simulink model "FilterDesigner"  (R2018b)
settings: Solver=VariableStepAuto  StartTime=0.0  StopTime=4000  RelTol=1e-3
PreLoadFcn:
  | Init
StopFcn:
  | FilterCheck
values from neighbouring files (symbols this model uses):
  fc = 0.33    [Init.m]
  h_win = blackman(N)    [Init.m]
  N = 101    [Init.m]
  NFFT = 1024    [Init.m]
  output_wlength = 24    [Init.m]
undefined symbols (not defined in the file or in its folder): AXI4, bitrevorder, int, Lite
libraries: xbsIndex_r4 x64
settings Model: Creator=joshua goldsmith  LastModifiedBy=jng
settings DebuggingCC: LibraryContextMissingDiagnostic=none
settings SFSimCC: SimUseLocalCustomCode=off
settings RTWCC: RTWUseLocalCustomCode=off

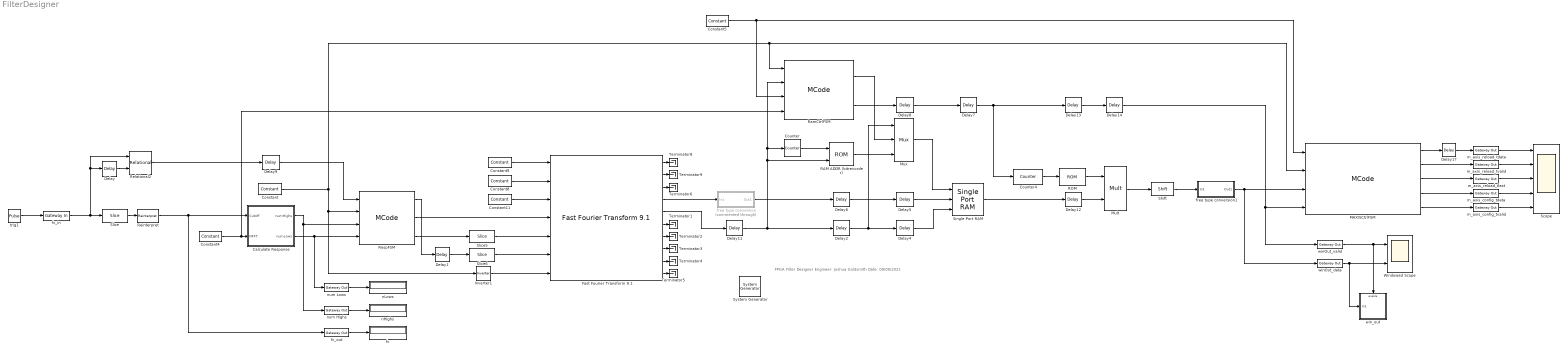
== system FilterDesigner ==
  note: FPGA Filter Designer
      | Engineer: Joshua Goldsmith
      | Date: 09/09/2021
  " System Generator" : xbsIndex_r4/ System Generator  Tag=genX  xilinxfamily=zynq  part=xc7z020  speed=-2  package=clg484  synthesis_tool=Vivado  clock_wrapper=Clock Enables  directory=./iprepo  proj_type=Vivado  Synth_file=Vivado Synthesis Defaults  Impl_file=Vivado Implementation Defaults  testbench=off  simulink_period=1  sysclk_period=10  dcm_input_clock_period=10  incr_netlist=off  trim_vbits=Everywhere in SubSystem  dbl_ovrd=According to Block Masks  core_generation=According to Block Masks  run_coregen=off  deprecated_control=off  eval_field=0  block_type=sysgen
  Calculate Response : Subsystem
  Constant : xbsIndex_r4/Constant  const=0  gui_display_data_type=Boolean  arith_type=Boolean  n_bits=16  bin_pt=14  preci_type=Single  exp_width=8  frac_width=24  explicit_period=on  period=1  equ=P=C  opselect=C  inp2=PCIN>>17  opr=+  inp1=P  carry=CIN  dbl_ovrd=off  block_type=constant
  Constant11 : xbsIndex_r4/Constant  const=0  gui_display_data_type=Fixed-point  arith_type=Signed (2's comp)  n_bits=wlength  bin_pt=flength  preci_type=Single  exp_width=8  frac_width=24  explicit_period=on  period=1  equ=P=C  opselect=C  inp2=PCIN>>17  opr=+  inp1=P  carry=CIN  dbl_ovrd=off  block_type=constant
  Constant4 : xbsIndex_r4/Constant  const=NFFT  gui_display_data_type=Fixed-point  arith_type=Unsigned  n_bits=log2(NFFT)+1  bin_pt=0  preci_type=Single  exp_width=8  frac_width=24  explicit_period=on  period=1  equ=P=C  opselect=C  inp2=PCIN>>17  opr=+  inp1=P  carry=CIN  dbl_ovrd=off  block_type=constant
  Constant5 : xbsIndex_r4/Constant  const=(N-1)/2  gui_display_data_type=Fixed-point  arith_type=Unsigned  n_bits=32  bin_pt=0  preci_type=Single  exp_width=8  frac_width=24  explicit_period=on  period=1  equ=P=C  opselect=C  inp2=PCIN>>17  opr=+  inp1=P  carry=CIN  dbl_ovrd=off  block_type=constant
  Constant8 : xbsIndex_r4/Constant  const=1  gui_display_data_type=Boolean  arith_type=Boolean  n_bits=wlength  bin_pt=flength  preci_type=Single  exp_width=8  frac_width=24  explicit_period=on  period=1  equ=P=C  opselect=C  inp2=PCIN>>17  opr=+  inp1=P  carry=CIN  dbl_ovrd=off  block_type=constant
  Constant9 : xbsIndex_r4/Constant  const=0  gui_display_data_type=Fixed-point  arith_type=Unsigned  n_bits=1  bin_pt=0  preci_type=Single  exp_width=8  frac_width=24  explicit_period=on  period=1  equ=P=C  opselect=C  inp2=PCIN>>17  opr=+  inp1=P  carry=CIN  dbl_ovrd=off  block_type=constant
  Counter : xbsIndex_r4/Counter  cnt_type=Free Running  cnt_to=Inf  operation=Up  start_count=0  cnt_by_val=1  arith_type=Unsigned  n_bits=log2(NFFT)  bin_pt=0  load_pin=off  rst=off  en=on  explicit_period=on  period=1  use_behavioral_HDL=off  implementation=Fabric  dbl_ovrd=off  block_type=counter
  Counter4 : xbsIndex_r4/Counter  cnt_type=Count Limited  cnt_to=size(h_win(1:size(h_win,1)/2+1),1)-1  operation=Up  start_count=0  cnt_by_val=1  arith_type=Unsigned  n_bits=ceil(log2(N/2))  bin_pt=0  load_pin=off  rst=off  en=on  explicit_period=on  period=1  use_behavioral_HDL=off  implementation=Fabric  dbl_ovrd=off  block_type=counter
  Delay{,2,4,6..8,11..14,17} (11 alike) : xbsIndex_r4/Delay  rst=off  infoeditControl=Selection of Reset will increase slice count due to use of real FFs and instead of SRLs  en=off  latency=1  reg_retiming=off  dbl_ovrd=off  block_type=delay
  Delay1 : xbsIndex_r4/Delay  rst=off  infoeditControl=Selection of Reset will increase slice count due to use of real FFs and instead of SRLs  en=off  latency=NFFT-1  reg_retiming=off  dbl_ovrd=off  block_type=delay
  Delay5 : xbsIndex_r4/Delay  rst=off  infoeditControl=Selection of Reset will increase slice count due to use of real FFs and instead of SRLs  en=off  latency=2  reg_retiming=off  dbl_ovrd=off  block_type=delay
  Delay9 : xbsIndex_r4/Delay  rst=off  infoeditControl=Selection of Reset will increase slice count due to use of real FFs and instead of SRLs  en=off  latency=3  reg_retiming=off  dbl_ovrd=off  block_type=delay
  "Fast Fourier Transform 9.1 " : xbsIndex_r4/Fast Fourier Transform 9.1   transform_length=1024  target_clock_frequency=100  target_data_throughput=50  implementation_options=pipelined_streaming_io  run_time_configurable_transform_length=off  phase_factor_width=16  scaling_options=unscaled  rounding_modes=truncation  aclken=off  aresetn=on  output_ordering=bit_reversed_order  cyclic_prefix_insertion=off  throttle_scheme=realtime  xk_index=off  ovflo=off  trim_axipin_name=on  memory_options_data=block_ram  memory_options_phase_factors=block_ram  number_of_stages_using_block_ram_for_data_and_phase_factors=2  memory_options_reorder=block_ram  memory_options_hybrid=off  complex_mult_type=use_mults_resources  butterfly_type=use_luts  simulation_type=hybrid_sim  simulation_model=sysgen:xfftv9_cmodel  data_path_portlist={ 's_axis_data_tdata', 'm_axis_data_tdata', 'm_axis_status_tdata', 'event_fft_overflow' }  channels=1  input_ordering=natural_order  input_width=16  ip_name=Fast Fourier Transform  ip_version=9.1  dsptool_ready=true  ipcore_usecache=true  ipcore_useipmodelcache=true  wrapper_available=true  port_translation_map={ 'aclken' => 'en', 'aresetn' => 'rst'}  data_format=fixed_point  block_type=xfft_v9_1
  Inverter1 : xbsIndex_r4/Inverter  en=off  latency=0  dbl_ovrd=off  block_type=inv
  MAXISCtrlFSM : xbsIndex_r4/MCode  mfname=MAXISCtrlFSM  explicit_period=on  period=1  inputsTable={'boundInpExpr'=>['',''],'inputs'=>['x','y']}  outputsTable={'outputs'=>['z'],'suppressOut'=>['off']}  enable_stdout=off  enable_debug=off  suppress_output=on  defparams={}  hide_port_list={}  dbl_ovrd=off  block_type=mcode
  Mult : xbsIndex_r4/Mult  precision=Full  arith_type="Signed  (2's comp)"  n_bits=16  bin_pt=14  quantization=Truncate  overflow=Wrap  en=off  latency=1  use_behavioral_HDL=off  opt=Speed  use_embedded=on  optimum_pipeline=off  pipeline=on  dbl_ovrd=off  use_rpm=on  placement_style=Triangular  block_type=mult
  Mux : xbsIndex_r4/Mux  inputs=2  en=off  latency=1  precision=Full  arith_type=Unsigned  n_bits=16  bin_pt=14  quantization=Truncate  overflow=Wrap  dbl_ovrd=off  block_type=mux
  RAM ADDR (bitrevorder) : xbsIndex_r4/ROM  depth=NFFT  initVector=bitrevorder(0:NFFT-1)  distributed_mem=Block RAM  rst=off  init_reg=0  en=on  latency=1  gui_display_data_type=Fixed-point  arith_type=Unsigned  n_bits=log2(NFFT)  bin_pt=0  preci_type=Single  exp_width=8  frac_width=24  optimize=Area  use_rpm=on  dbl_ovrd=off  block_type=sprom
  ROM : xbsIndex_r4/ROM  depth=(N+1)/2  initVector=h_win(1:size(h_win,1)/2+1)  distributed_mem=Block RAM  rst=off  init_reg=0  en=off  latency=1  gui_display_data_type=Fixed-point  arith_type="Signed  (2's comp)"  n_bits=16  bin_pt=14  preci_type=Single  exp_width=8  frac_width=24  optimize=Area  use_rpm=on  dbl_ovrd=off  block_type=sprom
  RamCtrlFSM : xbsIndex_r4/MCode  mfname=RamCtrlFSM  explicit_period=on  period=1  inputsTable={'boundInpExpr'=>['','','','',''],'inputs'=>['rst','valid_in','M','NFFT','wlength']}  outputsTable={'outputs'=>['addr','valid_out'],'suppressOut'=>['off','off']}  enable_stdout=off  enable_debug=off  suppress_output=on  defparams={}  hide_port_list={}  dbl_ovrd=off  block_type=mcode
  Reinterpret : xbsIndex_r4/Reinterpret  force_arith_type=on  arith_type=Unsigned  force_bin_pt=on  bin_pt=10  block_type=reinterpret
  Relational2 : xbsIndex_r4/Relational  mode=a!=b  op_type=Bool  en=off  latency=0  dbl_ovrd=off  block_type=relational
  RespFSM : xbsIndex_r4/MCode  mfname=RespFSM  explicit_period=on  period=1  inputsTable={'boundInpExpr'=>['','','',''],'inputs'=>['trig','rst','numHighs','numLows']}  outputsTable={'outputs'=>['sof','rout','valid'],'suppressOut'=>['off','off','off']}  enable_stdout=off  enable_debug=off  suppress_output=on  defparams={}  hide_port_list={}  dbl_ovrd=off  block_type=mcode
  Scope : Scope  NumInputPorts=5
  Shift : xbsIndex_r4/Shift  shift_dir=Left  shift_bits=3  en=off  latency=0  precision=Full  arith_type="Signed  (2's comp)"  n_bits=16  bin_pt=14  quantization=Truncate  overflow=Wrap  dbl_ovrd=off  block_type=shift
  Single Port RAM : xbsIndex_r4/Single Port RAM  depth=NFFT  initVector=zeros(1,NFFT)  distributed_mem=Block RAM  write_mode=No Read On Write  rst=off  init_reg=0  en=off  latency=1  optimize=Area  dbl_ovrd=off  block_type=spram
  Slice : xbsIndex_r4/Slice  nbits=10  boolean_output=off  mode=Lower Bit Location + Width  bit1=0  base1=MSB of Input  bit0=0  base0=LSB of Input  dbl_ovrd=off  block_type=slice
  Slice5 : xbsIndex_r4/Slice  nbits=1  boolean_output=on  mode=Lower Bit Location + Width  bit1=0  base1=MSB of Input  bit0=0  base0=LSB of Input  dbl_ovrd=off  block_type=slice
  Slice6 : xbsIndex_r4/Slice  nbits=1  boolean_output=on  mode=Lower Bit Location + Width  bit1=0  base1=MSB of Input  bit0=0  base0=LSB of Input  dbl_ovrd=off  block_type=slice
  Terminator{1..6,8..9} (8 alike) : Terminator
  Windowed Scope : Scope  NumInputPorts=2
  fc : Display
  fc_in : xbsIndex_r4/Gateway In  gui_display_data_type=Fixed-point  arith_type=Unsigned  n_bits=32  bin_pt=0  preci_type=Single  exp_width=8  frac_width=24  rows=1  columns=1  quantization=Truncate  overflow=Wrap  period=1  UseAsADC=off  ADCChannel='1'  interface=AXI4-Lite  automatic_assignment=off  address_offset=12  intf_name=''  intf_description=''  default_value=0  timing_constraint=None  locs_specified=off  LOCs={}  io_standard={}  inherit_from_input=off  hdl_port=on  dbl_ovrd=off  block_type=gatewayin
  fc_out : xbsIndex_r4/Gateway Out  inherit_from_input=off  hdl_port=off  rows=1  columns=1  UseAsDAC=off  DACChannel='1'  interface=None  automatic_assignment=on  address_offset=hex2dec('00')  intf_name=''  intf_description=''  timing_constraint=None  locs_specified=off  LOCs={}  io_standard={}  block_type=gatewayout
  free type conversion : Subsystem  Commented=through  mask{Wordlength=16, FracBit=15}
      mask prompts: FracBit "Fractional Bit Position"
      mask DialogControl DescGroupVar Prompt: Type Conversion
      mask DialogControl DescTextVar Prompt: Select wordlength and fractional bit position
  free type conversion1 : Subsystem  mask{Wordlength=output_wlength, FracBit=output_wlength-1}
      mask prompts: FracBit "Fractional Bit Position"
      mask DialogControl DescGroupVar Prompt: Type Conversion
      mask DialogControl DescTextVar Prompt: Select wordlength and fractional bit position
  m_axis_config_tdata : xbsIndex_r4/Gateway Out  inherit_from_input=off  hdl_port=on  rows=1  columns=1  UseAsDAC=off  DACChannel='1'  interface=None  automatic_assignment=on  address_offset=hex2dec('00')  intf_name=''  intf_description=''  timing_constraint=None  locs_specified=off  LOCs={}  io_standard={}  block_type=gatewayout
  m_axis_config_tvalid : xbsIndex_r4/Gateway Out  inherit_from_input=off  hdl_port=on  rows=1  columns=1  UseAsDAC=off  DACChannel='1'  interface=None  automatic_assignment=on  address_offset=hex2dec('00')  intf_name=''  intf_description=''  timing_constraint=None  locs_specified=off  LOCs={}  io_standard={}  block_type=gatewayout
  m_axis_reload_tdata : xbsIndex_r4/Gateway Out  inherit_from_input=off  hdl_port=on  rows=1  columns=1  UseAsDAC=off  DACChannel='1'  interface=None  automatic_assignment=on  address_offset=hex2dec('00')  intf_name=''  intf_description=''  timing_constraint=None  locs_specified=off  LOCs={}  io_standard={}  block_type=gatewayout
  m_axis_reload_tlast : xbsIndex_r4/Gateway Out  inherit_from_input=off  hdl_port=on  rows=1  columns=1  UseAsDAC=off  DACChannel='1'  interface=None  automatic_assignment=on  address_offset=hex2dec('00')  intf_name=''  intf_description=''  timing_constraint=None  locs_specified=off  LOCs={}  io_standard={}  block_type=gatewayout
  m_axis_reload_tvalid : xbsIndex_r4/Gateway Out  inherit_from_input=off  hdl_port=on  rows=1  columns=1  UseAsDAC=off  DACChannel='1'  interface=None  automatic_assignment=on  address_offset=hex2dec('00')  intf_name=''  intf_description=''  timing_constraint=None  locs_specified=off  LOCs={}  io_standard={}  block_type=gatewayout
  nHighs : Display
  nLows : Display
  "num Highs " : xbsIndex_r4/Gateway Out  inherit_from_input=off  hdl_port=off  rows=1  columns=1  UseAsDAC=off  DACChannel='1'  interface=None  automatic_assignment=on  address_offset=hex2dec('00')  intf_name=''  intf_description=''  timing_constraint=None  locs_specified=off  LOCs={}  io_standard={}  block_type=gatewayout
  "num Lows " : xbsIndex_r4/Gateway Out  inherit_from_input=off  hdl_port=off  rows=1  columns=1  UseAsDAC=off  DACChannel='1'  interface=None  automatic_assignment=on  address_offset=hex2dec('00')  intf_name=''  intf_description=''  timing_constraint=None  locs_specified=off  LOCs={}  io_standard={}  block_type=gatewayout
  trig1 : DiscretePulseGenerator  Amplitude=int(fi(fc,0,10,10))  Period=5000  PulseWidth=5000
  winOut_data : xbsIndex_r4/Gateway Out  inherit_from_input=off  hdl_port=off  rows=1  columns=1  UseAsDAC=off  DACChannel='1'  interface=None  automatic_assignment=on  address_offset=hex2dec('00')  intf_name=''  intf_description=''  timing_constraint=None  locs_specified=off  LOCs={}  io_standard={}  block_type=gatewayout
  winOut_valid : xbsIndex_r4/Gateway Out  inherit_from_input=off  hdl_port=off  rows=1  columns=1  UseAsDAC=off  DACChannel='1'  interface=None  automatic_assignment=on  address_offset=hex2dec('00')  intf_name=''  intf_description=''  timing_constraint=None  locs_specified=off  LOCs={}  io_standard={}  block_type=gatewayout
  win_out : Subsystem
  wires:
  Constant4/1 -> RamCtrlFSM/4, Calculate Response/2(NFFT)
  Calculate Response/2(numLows) -> "num Lows "/1, RespFSM/4
  Calculate Response/1(numHighs) -> RespFSM/3, "num Highs "/1
  RespFSM/3 -> Slice5/1
  RespFSM/2 -> "Fast Fourier Transform 9.1 "/4
  RespFSM/1 -> Delay1/1
  Constant/1 -> MAXISCtrlFSM/2, RamCtrlFSM/1, Inverter1/1, RespFSM/2
  RAM ADDR (bitrevorder)/1 -> Mux/3
  Mux/1 -> Single Port RAM/1
  Delay5/1 -> Single Port RAM/2
  "num Highs "/1 -> nHighs/1
  "num Lows "/1 -> nLows/1
  Delay9/1 -> RespFSM/1
  Counter/1 -> RAM ADDR (bitrevorder)/1
  Delay2/1 -> Delay4/1, Mux/1
  Delay4/1 -> Single Port RAM/3
  Delay6/1 -> Delay5/1
  RamCtrlFSM/2 -> Delay8/1
  Delay8/1 -> Delay7/1
  free type conversion/1(Out1) -> Delay6/1
  Single Port RAM/1 -> Delay12/1
  ROM/1 -> Mult/1
  Delay12/1 -> Mult/2
  Delay13/1 -> Delay14/1
  winOut_valid/1 -> Windowed Scope/1, win_out/Enable
  winOut_data/1 -> win_out/1(In1), Windowed Scope/2
  MAXISCtrlFSM/2 -> m_axis_reload_tvalid/1
  MAXISCtrlFSM/3 -> m_axis_reload_tlast/1
  fc_out/1 -> fc/1
  MAXISCtrlFSM/4 -> m_axis_config_tdata/1
  MAXISCtrlFSM/5 -> m_axis_config_tvalid/1
  m_axis_reload_tlast/1 -> Scope/3
  m_axis_reload_tvalid/1 -> Scope/2
  m_axis_reload_tdata/1 -> Scope/1
  m_axis_config_tdata/1 -> Scope/4
  fc_in/1 -> Relational2/1, Delay/1, Slice/1
  Slice/1 -> Reinterpret/1
  MAXISCtrlFSM/1 -> Delay17/1
  Constant5/1 -> RamCtrlFSM/3, MAXISCtrlFSM/1
  Reinterpret/1 -> fc_out/1, Calculate Response/1(Cutoff)
  Delay14/1 -> winOut_valid/1, MAXISCtrlFSM/4
  RamCtrlFSM/1 -> Mux/2
  "Fast Fourier Transform 9.1 "/1 -> Terminator8/1
  "Fast Fourier Transform 9.1 "/2 -> Terminator9/1
  Slice5/1 -> "Fast Fourier Transform 9.1 "/5
  Slice6/1 -> "Fast Fourier Transform 9.1 "/6
  Delay1/1 -> Slice6/1
  Inverter1/1 -> "Fast Fourier Transform 9.1 "/7
  "Fast Fourier Transform 9.1 "/5 -> Delay11/1
  Delay11/1 -> Delay2/1, RAM ADDR (bitrevorder)/2, Counter/1, RamCtrlFSM/2
  Delay7/1 -> Delay13/1, Counter4/1
  Constant8/1 -> "Fast Fourier Transform 9.1 "/2
  Constant9/1 -> "Fast Fourier Transform 9.1 "/1
  Constant11/1 -> "Fast Fourier Transform 9.1 "/3
  Delay17/1 -> m_axis_reload_tdata/1
  Relational2/1 -> Delay9/1
  trig1/1 -> fc_in/1
  Delay/1 -> Relational2/2
  Mult/1 -> Shift/1
  Shift/1 -> free type conversion1/1(In1)
  free type conversion1/1(Out1) -> winOut_data/1, MAXISCtrlFSM/3
  "Fast Fourier Transform 9.1 "/4 -> free type conversion/1(In1)
  Counter4/1 -> ROM/1
  "Fast Fourier Transform 9.1 "/6 -> Terminator1/1
  "Fast Fourier Transform 9.1 "/7 -> Terminator2/1
  "Fast Fourier Transform 9.1 "/8 -> Terminator3/1
  "Fast Fourier Transform 9.1 "/9 -> Terminator4/1
  "Fast Fourier Transform 9.1 "/10 -> Terminator5/1
  "Fast Fourier Transform 9.1 "/3 -> Terminator6/1
  m_axis_config_tvalid/1 -> Scope/5

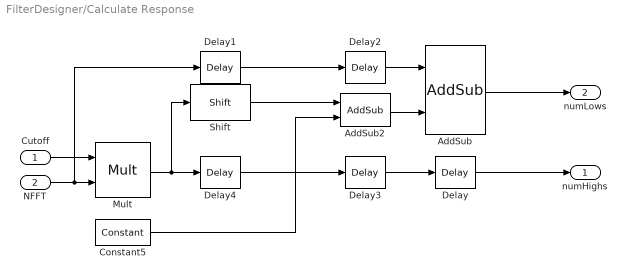
== system FilterDesigner/Calculate Response ==
  Cutoff : Inport
  NFFT : Inport  Port=2
  AddSub : xbsIndex_r4/AddSub  mode=Subtraction  use_carryin=off  use_carryout=off  en=off  latency=1  precision=User Defined  arith_type=Unsigned  n_bits=log2(NFFT)+1  bin_pt=0  quantization=Truncate  overflow=Wrap  use_behavioral_HDL=off  hw_selection=Fabric  pipelined=off  dbl_ovrd=off  block_type=addsub
  AddSub2 : xbsIndex_r4/AddSub  mode=Subtraction  use_carryin=off  use_carryout=off  en=off  latency=1  precision=User Defined  arith_type=Unsigned  n_bits=log2(NFFT)+1  bin_pt=0  quantization=Truncate  overflow=Wrap  use_behavioral_HDL=off  hw_selection=Fabric  pipelined=off  dbl_ovrd=off  block_type=addsub
  Constant5 : xbsIndex_r4/Constant  const=1.0  gui_display_data_type=Fixed-point  arith_type=Unsigned  n_bits=1  bin_pt=0  preci_type=Single  exp_width=8  frac_width=24  explicit_period=on  period=1  equ=P=C  opselect=C  inp2=PCIN>>17  opr=+  inp1=P  carry=CIN  dbl_ovrd=off  block_type=constant
  Delay{,2..4} (4 alike) : xbsIndex_r4/Delay  rst=off  infoeditControl=Selection of Reset will increase slice count due to use of real FFs and instead of SRLs  en=off  latency=1  reg_retiming=off  dbl_ovrd=off  block_type=delay
  Delay1 : xbsIndex_r4/Delay  rst=off  infoeditControl=Selection of Reset will increase slice count due to use of real FFs and instead of SRLs  en=off  latency=2  reg_retiming=off  dbl_ovrd=off  block_type=delay
  Mult : xbsIndex_r4/Mult  precision=User Defined  arith_type=Unsigned  n_bits=log2(NFFT)+1  bin_pt=0  quantization="Round  (unbiased: +/- Inf)"  overflow=Wrap  en=off  latency=1  use_behavioral_HDL=off  opt=Speed  use_embedded=on  optimum_pipeline=off  pipeline=on  dbl_ovrd=off  use_rpm=on  placement_style=Triangular  block_type=mult
  Shift : xbsIndex_r4/Shift  shift_dir=Left  shift_bits=1  en=off  latency=1  precision=Full  arith_type=Unsigned  n_bits=20  bin_pt=0  quantization="Round  (unbiased: +/- Inf)"  overflow=Wrap  dbl_ovrd=off  block_type=shift
  numHighs : Outport
  numLows : Outport  Port=2
  wires:
  AddSub/1 -> numLows/1
  NFFT/1 -> Delay1/1, Mult/2
  Mult/1 -> Delay4/1, Shift/1
  Cutoff/1 -> Mult/1
  Delay/1 -> numHighs/1
  Shift/1 -> AddSub2/1
  AddSub2/1 -> AddSub/2
  Delay1/1 -> Delay2/1
  Delay2/1 -> AddSub/1
  Delay3/1 -> Delay/1
  Delay4/1 -> Delay3/1
  Constant5/1 -> AddSub2/2

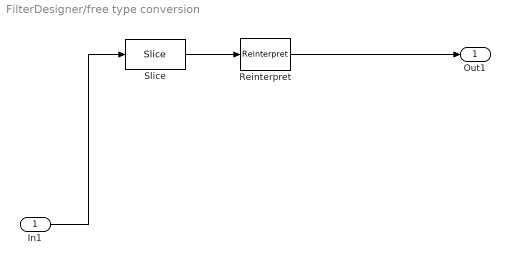
== system FilterDesigner/free type conversion ==
  In1 : Inport
  Reinterpret : xbsIndex_r4/Reinterpret  force_arith_type=on  arith_type="Signed  (2's comp)"  force_bin_pt=on  bin_pt=FracBit  block_type=reinterpret
  Slice : xbsIndex_r4/Slice  nbits=Wordlength  boolean_output=off  mode=Upper Bit Location + Width  bit1=0  base1=MSB of Input  bit0=0  base0=LSB of Input  dbl_ovrd=off  block_type=slice
  Out1 : Outport
  wires:
  Slice/1 -> Reinterpret/1
  In1/1 -> Slice/1
  Reinterpret/1 -> Out1/1

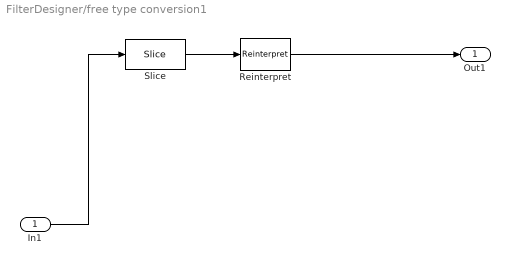
== system FilterDesigner/free type conversion1 ==
  In1 : Inport
  Reinterpret : xbsIndex_r4/Reinterpret  force_arith_type=on  arith_type="Signed  (2's comp)"  force_bin_pt=on  bin_pt=FracBit  block_type=reinterpret
  Slice : xbsIndex_r4/Slice  nbits=Wordlength  boolean_output=off  mode=Upper Bit Location + Width  bit1=0  base1=MSB of Input  bit0=0  base0=LSB of Input  dbl_ovrd=off  block_type=slice
  Out1 : Outport
  wires:
  Reinterpret/1 -> Out1/1
  In1/1 -> Slice/1
  Slice/1 -> Reinterpret/1

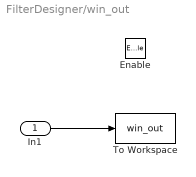
== system FilterDesigner/win_out ==
  In1 : Inport
  Enable : EnablePort
  To Workspace : ToWorkspace  VariableName=win_out  SampleTime=-1
      settings: Save2DSignal=2-D array (concatenate along first dimension)
  wires:
  In1/1 -> To Workspace/1
